simulink library "DKE_Library"  (R2018b)
settings: Solver=VariableStepAuto  StartTime=0.0  StopTime=10.0  RelTol=1e-3
undefined symbols (not defined in the file): dke, ENV, eta_panel, GM, GM_EARTH, Id, N_surf, P0_Sun, q0, r0, req_dke, RW, S_panels, S_surf, SC, v0, vf, w0, ww0, x0
libraries: MATH_library x18, ENV_Library x13, $bdroot x8, simulink x2, sharedtransform x1
(part 1 of 2)
settings Model: Creator=Andrea  LastModifiedBy=andrea

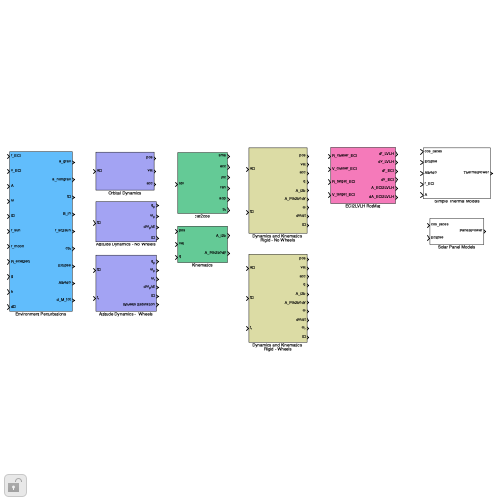
[thumbnail: Simulink's stored preview of the top-level diagram]
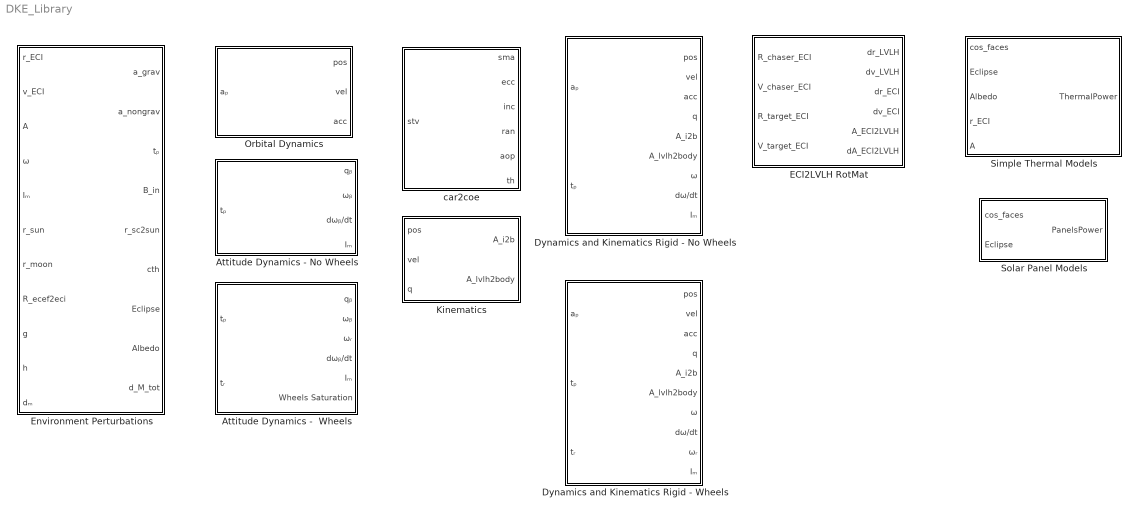
== system DKE_Library ==
  " Simple Thermal Models" : Subsystem  mask(Simple Thermal Modelling){P0_Sun=P0_Sun, BODY_RADIUS=req_dke, S_surf=S_surf, N_surf=N_surf, vf=vf}
      mask prompts: BODY_RADIUS "Earth Radius [m]:"; S_surf "Faces Areas [m²]:"; N_surf "Faces Normals:"; vf "View Factors Coefficients:"
      mask help:
      | Compute the thermal power acting on the spacecraft with a simple model.
      |
      | INPUTS:
      |   - Cosine of the angles between the surface normals and the sun direction.
      |   - Eclipse flag (1 = Eclipse ON)
      |   - Albedo falg (1 = Albedo ON)
      |   - Spacecraft Position in the Inertial Frame [m].
      |   - DCM from the inertial to the Principal Inertia Axes.
      |
      | CHANGELOG:
      |  - 2018: Andrea Colagrossi - First Release
      |  - 2023: Michele Ceresoli -  Polished
      mask DialogControl Container2 Prompt: Parameters
  Attitude Dynamics -  Wheels : Subsystem  mask(Rigid Attitude Dynamics - With Reaction Wheels){q0=q0, w0=w0, ww0=ww0, I=SC.I, invI=SC.invI, RW=RW}
      mask prompts: q0 "Initial Quaternion:"; w0 "Initial Angular Velocity [rad/s]:"; ww0 "Initial RW Angular Velocity [rad/s]"; I "Inertia Matrix [kgm²]:"; invI "Inverse Inertia Matrix [1/kgm²]"; RW "Reaction Wheels Structure:"
      mask help:
      | Integrate the controlled (with reaction wheels) attitude dynamics of a spacecraft without the flexibility and sloshing effects.
      |
      | INPUTS:
      |   - Perturbing torque [Nm]
      |   - Reaction wheels torque [Nm]
      |
      | OUTPUTS:
      |   - Quaternion from the inertial to the Principal Inertial Axes
      |   - Spacecraft angular velocity in the Principal Inertial Axes [rad/s]
      |   - Reaction wheels angular velocity [rad/s]
      |   - Angular velocity derivative in the Principal Inertial Axes [rad/s²]
      |   - Spacecraft inertia matrix [kgm²]
      |   - Wheels Saturation flag (true if saturated)
      |
      | CHANGELOG:
      |   - 2018: Andrea Colagrossi - First Release
      |   - 2023: Michele Ceresoli - Polished
      mask DialogControl Container2 Prompt: Parameters:
  Attitude Dynamics - No Wheels : Subsystem  mask(Rigid Attitude Dynamics - Without Reaction Wheels){q0=q0, w0=w0, I=SC.I, invI=SC.invI}
      mask prompts: q0 "Initial Quaternion:"; w0 "Initial Angular Velocity [rad/s]:"; I "Inertia Matrix [kgm²]:"; invI "Inverse Inertia Matrix [1/kgm²]"
      mask help:
      | Integrate the uncontrolled (no reaction wheels) attitude dynamics of a spacecraft without the flexibility and sloshing effects.
      |
      | INPUTS:
      |   - Perturbing torque [Nm]
      |
      | OUTPUTS:
      |   - Quaternion from the inertial to the Principal Inertial Axes
      |   - Spacecraft angular velocity in the Principal Inertial Axes [rad/s]
      |   - Angular velocity derivative in the Principal Inertial Axes [rad/s²]
      |   - Spacecraft inertia matrix [kgm²]
      |
      | CHANGELOG:
      |   - 2018: Andrea Colagrossi - First Release
      |   - 2023: Michele Ceresoli - Polished
      mask DialogControl Container2 Prompt: Parameters:
  Dynamics and Kinematics Rigid - No Wheels : Subsystem  mask(Rigid Dynamics and Kinematics - No Wheels){r0=r0, v0=v0, w0=w0, q0=q0, Im=SC, InvIm=SC, GM_BODY=0}
      mask prompts: r0 "Initial Position [m]:"; v0 "Initial Velocity [m/s]:"; w0 "Initial Angular velocity [rad/s]:"; q0 "Initial Quaternion:"; Im "Inertia Matrix [kgm²]"; InvIm "Inverse Inertia Matrix [1/kgm²]"; GM_BODY "Planetary Constant [m³/s²]"
      mask help:
      | Propagate the uncontrolled attitude dynamics and kinematics with a rigid model (no flexibility and sloshing).
      |
      | INPUTS:
      |   - Perturbing inertial acceleration [m/s²]
      |   - Perturbing torque in the PIA [Nm]
      |
      | OUTPUTS:
      |   - Inertial position [m]
      |   - Inertial velocity [m/s]
      |   - Inertial acceleration [m/s²]
      |   - Quaternion from the Inertial to the PIA
      |   - DCM from the Inertial to the PIA
      |   - DCM from the LVLH to the PIA
      |   - Angular velocity in the PIA [rad/s]
      |   - Angular velocity derivative in the PIA [rad/s²]
      |   - Inertia Matrix [kgm²]
      |
      | NOTES:
      |   - PIA stands for Principal Inertial Axes.
      |
      | CHANGELOG:
      |   - 2018: Andrea Colagrossi - First Release
      |   - 2023: Michele Ceresoli -  Rework, Tested and Polished
      mask DialogControl Container3 Prompt: Initial Conditions
      mask DialogControl Container4 Prompt: Properties
  Dynamics and Kinematics Rigid - Wheels : Subsystem  mask(Rigid Dynamics and Kinematics - Wheels){r0=r0, v0=v0, w0=w0, ww0=0, q0=q0, Im=SC, InvIm=ENV, GM_BODY=0, RWL=0}
      mask prompts: r0 "Initial position [m]:"; v0 "Initial velocity [m/s]:"; w0 "Initial angular velocity [rad/s]:"; ww0 "RW Initial angular velocity [rad/s]"; q0 "Initial quaternion:"; Im "Inertia Matrix [kgm²]"; InvIm "Inverse Inertia Matrix [1/kgm²]"; GM_BODY "Planetary Constant [m³/s²]"; RWL "Reaction Wheels structure"
      mask help:
      | Propagate the attitude dynamics and kinematics with a rigid model (no flexibility and sloshing) including the reaction wheels control.
      |
      | INPUTS:
      |   - Perturbing inertial acceleration [m/s²]
      |   - Perturbing torque in the PIA [Nm]
      |
      | OUTPUTS:
      |   - Inertial position [m]
      |   - Inertial velocity [m/s]
      |   - Inertial acceleration [m/s²]
      |   - Quaternion from the Inertial to the PIA
      |   - DCM from the Inertial to the PIA
      |   - DCM from the LVLH to the PIA
      |   - Angular velocity in the PIA [rad/s]
      |   - Angular velocity derivative in the PIA [rad/s²]
      |   - Reaction wheels angular velocity [rad/s]
      |   - Inertia Matrix [kgm²]
      |
      | NOTES:
      |   - PIA stands for Principal Inertial Axes.
      |
      | CHANGELOG:
      |   - 2018: Andrea Colagrossi - First Release
      |   - 2023: Michele Ceresoli -  Rework, Tested and Polished
      mask DialogControl Container3 Prompt: Initial Conditions
      mask DialogControl Container4 Prompt: Properties
  ECI2LVLH RotMat : Subsystem  mask(ECI2LVLH Rotation Block){ref_obj=1, GM=dke.GM_EARTH}
      mask prompts: ref_obj "Reference LVLH object (1 for chaser, -1 for target)"; GM "Gravitational constant [m³/s²]:"
      mask help:
      | © ASTRA - Aerospace Science and Technology Dept. - PoliMi - 2023
      |
      | Relative position and velocity rotation ECI to/from LVLH.
      |
      | Input and output in SI units [m, m/s].
      mask DialogControl Container2 Prompt: Parameters:
  Environment Perturbations : Subsystem  mask(Environment Perturbations){GM_EARTH=ENV.GM_EARTH, GM_MOON=ENV.GM_MOON, GM_SUN=ENV.GM_SUN, RADIUS_EARTH=ENV.RADIUS_EARTH, RADIUS_SUN=ENV.RADIUS_SUN, ATMO_HEIGHT=0, mag_data=ENV.mag_data, grav_data=ENV.grav_data, rho_h=ENV.rho_h, NS=SC.NS, S_faces=SC.S_surf, N_faces=SC.N_surf, R_faces=SC.R_surf, c_dif=SC.c_dif, c_spe=SC.c_spe, CD=SC.C_D, mass=SC.m_sc, paras_dipole=SC.d, Keddy=SC.Keddy}
      mask prompts: GM_EARTH "Earth's Gravitational Constant [m³/s²]:"; GM_MOON "Moon's Gravitational Constant [m³/s²]:"; GM_SUN "Sun's Gravitational Constant [m³/s²]:"; RADIUS_EARTH "Earth's Radius [m]"; RADIUS_SUN "Sun's Radius [m]"; ATMO_HEIGHT "Earth's Atmosphere Height [m]"; mag_data "Magnetic Field Data:"; grav_data "Gravity Field Data:"; rho_h "Air Density Data:"; NS "Number of Faces"; S_faces "Faces Areas [m²]:"; N_faces "Faces Normals:"; R_faces "Faces Center of Pressures wrt CoM [m]:"; c_dif "Diffuse Coefficient [-]:"; c_spe "Specular Coefficient [-]:"; CD "Drag Coefficient [-]:"; mass "Mass [kg]:"; paras_dipole "Parasitic Magnetic Dipole [Am²]:"; Keddy "Eddy Currents Coefficient []:"
      mask help:
      | Compute the environment perturbing acceleration [m/s²] and torque [Nm] that act on a spacecraft. The perturbations include:
      |   - Moon's gravity
      |   - Sun's gravity
      |   - Earth's spherical harmonics
      |   - Gravity gradient torque
      |   - SRP acceleration and torque (with the plate model)
      |   - Drag acceleration and torque (with the plate model)
      |   - Magnetic torque (dipole and Eddy currents)
      |
      | INPUTS:
      |   - r_ECI, v_ECI: Spacecraft positions in the ECI frame [m]
      |   - A: DCM from the inertial to the Principal Inertia Frame
      |   - ω: Spacecraft angular velocity in the Principal Inertia Frame [rad/s]
      |   - Iₘ: Spacecraft Inertia Matrix [kgm²]
      |   - TT: Terrestrial time seconds since J2000
      |   - r_sun, r_moon: Sun's and Moon's positions in the ECI frame [m]
      |   - R_ecef2eci: ECEF to ECI rotation matrix
      |   - g, h: Magnetic Field coefficients at epoch.
      |   - dₘ: Magnetorquer Magnetic Dipole [Am²]
      |
      | NOTES:
      |   - A simple atmospheric model is used to compute the air density.
      |   - The gravity field data is extracted from the "load_gravity_model" function.
      |   - All the inputs and outputs are expressed in SI units (m, m/s, rad/s, kg, T, etc..).
      |
      | CHANGELOG:
      |   - 2018: Andrea Colagrossi - First Release
      |   - 2023: Michele Ceresoli - Rework, Testing and Polishing
      mask DialogControl Container3 Prompt: Environment:
      mask DialogControl Container4 Prompt: Spacecraft Geometry
      mask DialogControl Container5 Prompt: Spacecraft Properties
  Kinematics : Subsystem  mask(Kinematics){GM_BODY=0}
      mask prompts: GM_BODY "Planetary Gravitational Constant [m³/s²]:"
      mask help:
      | Compute the LVLH to Body and Inertial to Body 3x3 rotation matrices.
      |
      | INPUTS:
      |   - Attitude quaternion from the inertial to the body frame.
      |   - Inertial position [m]
      |   - Inertial velocity [m/s]
      |
      | CHANGELOG:
      |   - 2018: Andrea Colagrossi/Lorenzo Bucci - First Release
      |   - 2023: Michele Ceresoli - Reworked, Tested and Polished
  Orbital Dynamics : Subsystem  mask(Orbital Dynamics){r0=x0, v0=v0, GM=GM}
      mask prompts: r0 "Initial Position [m]:"; v0 "Initial Velocity [m/s]:"; GM "Central Body Gravitational Constant [m³/s²]:"
      mask help:
      | Propagate the spacecraft orbital dynamics by including the input perturbing acceleration to the two-body gravitational acceleration.
      |
      | INPUTS:
      |  - Perturbing acceleration [m/s²]
      |
      | OUTPUTS:
      |  - Inertial Position [m]
      |  - Inertial Velocity [m/s]
      |  - Inertial Acceleration [m/s²]
      |
      | CHANGELOG:
      |  - 2018: Andrea Colagrossi - First Release
      |  - 2023: Michele Ceresoli - Testing and Polishing
  Solar Panel Models : Subsystem  mask{P0_Sun=P0_Sun, eta_panel=eta_panel, Id=Id, S_panels=S_panels}
      mask help:
      | © Andrea Colagrossi - Aerospace Science and Technology Dept. - PoliMi - 2018
      |
      | Panels Electric Modelling
      |
      | Input and output in SI units [m, m/s, rad/s, kg, T, etc.]
      |
      | Cos_faces: Cosine of the Sun on Spacecraft Surfaces
      | Eclipse: Flag of the Eclipse Status (1 = Eclipse ON)
  car2coe : Subsystem  mask(Cartesian to Classical Orbital Elements (COE)){GM=GM_EARTH}
      mask prompts: GM "Planetary Gravitational Constant:"
      mask help: Convert a Cartesian state (position and velocity) to the Classical Orbital Elements (COE).

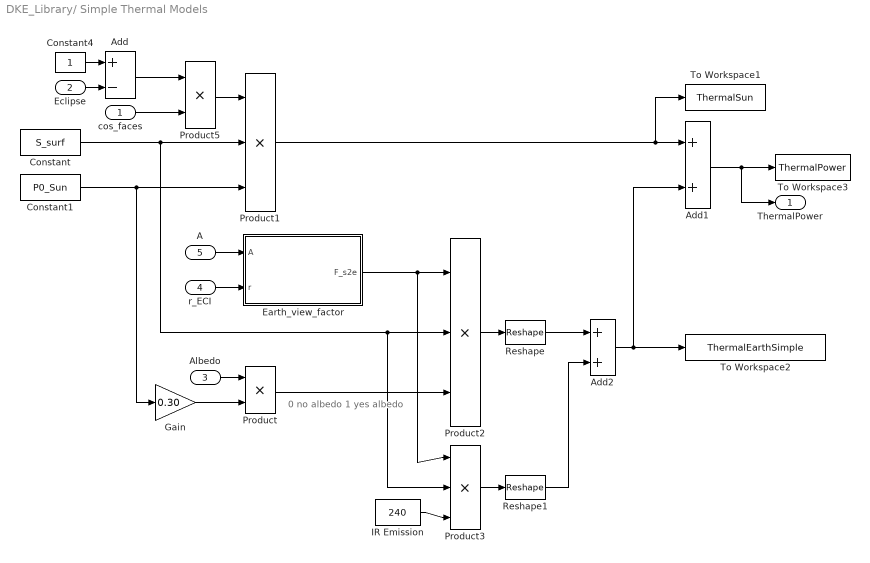
== system DKE_Library/ Simple Thermal Models ==
  note: 0 no albedo
      | 1 yes albedo
  cos_faces : Inport
  Eclipse : Inport  Port=2
  Albedo : Inport  Port=3
  r_ECI : Inport  Port=4
  A : Inport  Port=5
  Add : Sum  Inputs=+-
  Add1 : Sum
  Add2 : Sum
  Constant : Constant  Value=S_surf
  Constant1 : Constant  Value=P0_Sun
  Constant4 : Constant
  "Earth_view_factor " : Subsystem
  Gain : Gain  Gain=0.30
  IR Emission : Constant  Value=240
  Product : Product
  Product1 : Product  Inputs=3
  Product2 : Product  Inputs=3
  Product3 : Product  Inputs=3
  Product5 : Product
  Reshape : Reshape
  Reshape1 : Reshape
  To Workspace1 : ToWorkspace  VariableName=ThermalSun  SampleTime=-1
  To Workspace2 : ToWorkspace  VariableName=ThermalEarthSimple  SampleTime=-1
  To Workspace3 : ToWorkspace  VariableName=ThermalPower  SampleTime=-1
  ThermalPower : Outport  VectorParamsAs1DForOutWhenUnconnected=off
  wires:
  Gain/1 -> Product/2
  Albedo/1 -> Product/1
  Product/1 -> Product2/3
  IR Emission/1 -> Product3/3
  Constant1/1 -> Product1/3, Gain/1
  Product1/1 -> To Workspace1/1, Add1/1
  Product3/1 -> Reshape1/1
  Product2/1 -> Reshape/1
  Product5/1 -> Product1/1
  Eclipse/1 -> Add/2
  Constant4/1 -> Add/1
  cos_faces/1 -> Product5/2
  Add/1 -> Product5/1
  Constant/1 -> Product1/2, Product3/2, Product2/2
  Add2/1 -> To Workspace2/1, Add1/2
  Reshape/1 -> Add2/1
  Reshape1/1 -> Add2/2
  "Earth_view_factor "/1(F_s2e) -> Product2/1, Product3/1
  A/1 -> "Earth_view_factor "/1(A)
  r_ECI/1 -> "Earth_view_factor "/2("r ")
  Add1/1 -> ThermalPower/1, To Workspace3/1

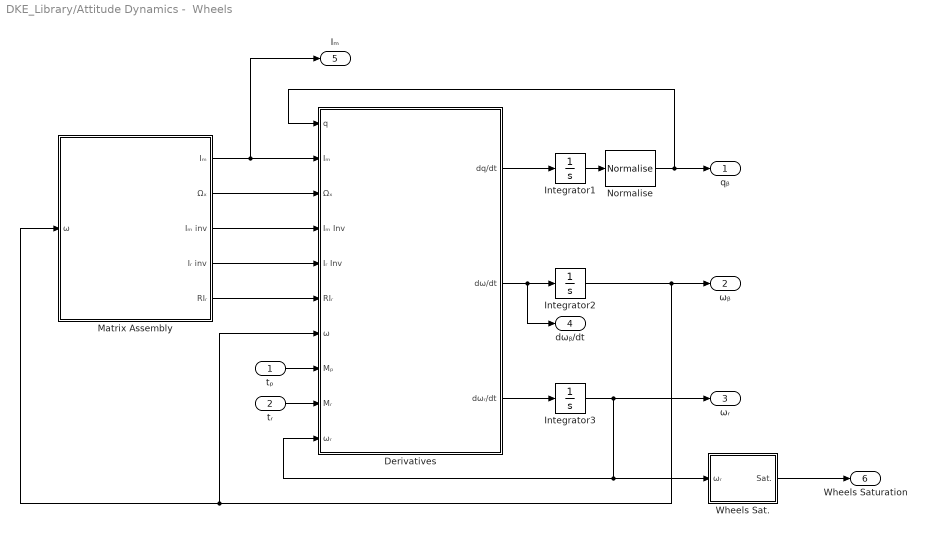
== system DKE_Library/Attitude Dynamics -  Wheels ==
  tₚ : Inport
  tᵣ : Inport  Port=2
  Derivatives : Subsystem
  Integrator1 : Integrator  InitialCondition=q0
  Integrator2 : Integrator  InitialCondition=w0
  Integrator3 : Integrator  InitialCondition=ww0  LimitOutput=on  UpperSaturationLimit=RW.MaxWheelW  LowerSaturationLimit=-RW.MaxWheelW
  Matrix Assembly : Subsystem
  Normalise : MATH_library/Normalise
  Wheels Sat. : Subsystem
  qᵦ : Outport  VectorParamsAs1DForOutWhenUnconnected=off
  ωᵦ : Outport  Port=2  VectorParamsAs1DForOutWhenUnconnected=off
  ωᵣ : Outport  Port=3  VectorParamsAs1DForOutWhenUnconnected=off
  dωᵦ/dt : Outport  Port=4  VectorParamsAs1DForOutWhenUnconnected=off
  Iₘ : Outport  Port=5  VectorParamsAs1DForOutWhenUnconnected=off
  Wheels Saturation : Outport  Port=6  VectorParamsAs1DForOutWhenUnconnected=off
  wires:
  Matrix Assembly/3(Iₘ inv) -> Derivatives/4(Iₘ Inv)
  Derivatives/2(dω/dt) -> dωᵦ/dt/1, Integrator2/1
  tₚ/1 -> Derivatives/8(Mₚ)
  Integrator2/1 -> ωᵦ/1, Derivatives/7(ω), Matrix Assembly/1("ω ")
  Matrix Assembly/1("Iₘ ") -> Derivatives/2(Iₘ), Iₘ/1
  Matrix Assembly/2(Ωₓ) -> Derivatives/3(Ωₓ)
  Derivatives/1(dq/dt) -> Integrator1/1
  Integrator1/1 -> Normalise/1
  Normalise/1 -> qᵦ/1, Derivatives/1(q)
  tᵣ/1 -> Derivatives/9(Mᵣ)
  Matrix Assembly/5(RIᵣ) -> Derivatives/6(RIᵣ)
  Matrix Assembly/4(Iᵣ inv) -> Derivatives/5(Iᵣ Inv)
  Derivatives/3(dωᵣ/dt) -> Integrator3/1
  Integrator3/1 -> Wheels Sat./1(ωᵣ), Derivatives/10(ωᵣ), ωᵣ/1
  Wheels Sat./1(Sat.) -> Wheels Saturation/1

== system DKE_Library/Attitude Dynamics - No Wheels ==
  tₚ : Inport
  Derivatives : Subsystem
  Integrator1 : Integrator  InitialCondition=q0
  Integrator2 : Integrator  InitialCondition=w0
  Matrix Assembly : Subsystem
  Normalise : MATH_library/Normalise
  qᵦ : Outport  VectorParamsAs1DForOutWhenUnconnected=off
  ωᵦ : Outport  Port=2  VectorParamsAs1DForOutWhenUnconnected=off
  dωᵦ/dt : Outport  Port=3  VectorParamsAs1DForOutWhenUnconnected=off
  Iₘ : Outport  Port=4  VectorParamsAs1DForOutWhenUnconnected=off
  wires:
  Matrix Assembly/3(Iₘ inv) -> Derivatives/4(Iₘ Inv)
  Derivatives/2(dω/dt) -> dωᵦ/dt/1, Integrator2/1
  tₚ/1 -> Derivatives/6(tₚ)
  Integrator2/1 -> ωᵦ/1, Derivatives/5(ω), Matrix Assembly/1("ω ")
  Matrix Assembly/1("Iₘ ") -> Iₘ/1, Derivatives/2(Iₘ)
  Matrix Assembly/2(Ωₓ) -> Derivatives/3(Ωₓ)
  Derivatives/1(dq/dt) -> Integrator1/1
  Integrator1/1 -> Normalise/1
  Normalise/1 -> qᵦ/1, Derivatives/1(q)

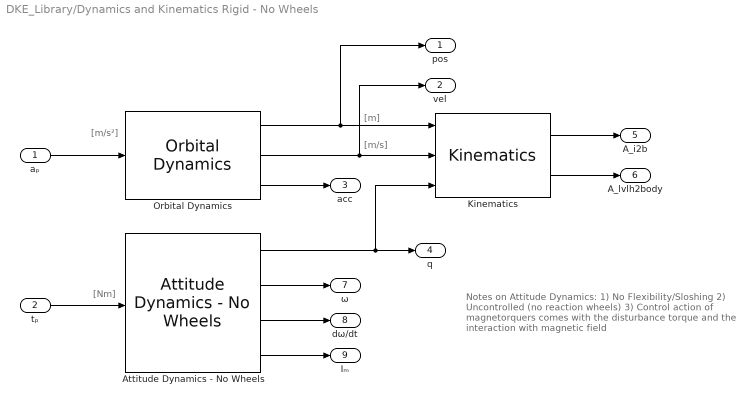
== system DKE_Library/Dynamics and Kinematics Rigid - No Wheels ==
  note: [m/s²]
  note: [Nm]
  note: [m]
  note: [m/s]
  note: Notes on Attitude Dynamics:
      | 1) No Flexibility/Sloshing
      | 2) Uncontrolled (no reaction wheels)
      | 3) Control action of magnetorquers comes with the disturbance torque and the interaction with magnetic field
  aₚ : Inport
  tₚ : Inport  Port=2
  Attitude Dynamics - No Wheels : $bdroot/Attitude Dynamics - No Wheels  q0=q0  w0=w0  I=Im  invI=InvIm
  Kinematics : $bdroot/Kinematics  GM_BODY=GM_BODY
  Orbital Dynamics : $bdroot/Orbital Dynamics  r0=r0  v0=v0  GM=GM_BODY
  pos : Outport  VectorParamsAs1DForOutWhenUnconnected=off
  vel : Outport  Port=2  VectorParamsAs1DForOutWhenUnconnected=off
  acc : Outport  Port=3  VectorParamsAs1DForOutWhenUnconnected=off
  q : Outport  Port=4  VectorParamsAs1DForOutWhenUnconnected=off
  A_i2b : Outport  Port=5  VectorParamsAs1DForOutWhenUnconnected=off
  A_lvlh2body : Outport  Port=6  VectorParamsAs1DForOutWhenUnconnected=off
  ω : Outport  Port=7  VectorParamsAs1DForOutWhenUnconnected=off
  dω/dt : Outport  Port=8  VectorParamsAs1DForOutWhenUnconnected=off
  Iₘ : Outport  Port=9  VectorParamsAs1DForOutWhenUnconnected=off
  wires:
  Orbital Dynamics/1 -> pos/1, Kinematics/1
  aₚ/1 -> Orbital Dynamics/1
  Kinematics/1 -> A_i2b/1
  Attitude Dynamics - No Wheels/1 -> q/1, Kinematics/3
  Orbital Dynamics/2 -> vel/1, Kinematics/2
  Orbital Dynamics/3 -> acc/1
  Attitude Dynamics - No Wheels/2 -> ω/1
  Kinematics/2 -> A_lvlh2body/1
  tₚ/1 -> Attitude Dynamics - No Wheels/1
  Attitude Dynamics - No Wheels/3 -> dω/dt/1
  Attitude Dynamics - No Wheels/4 -> Iₘ/1

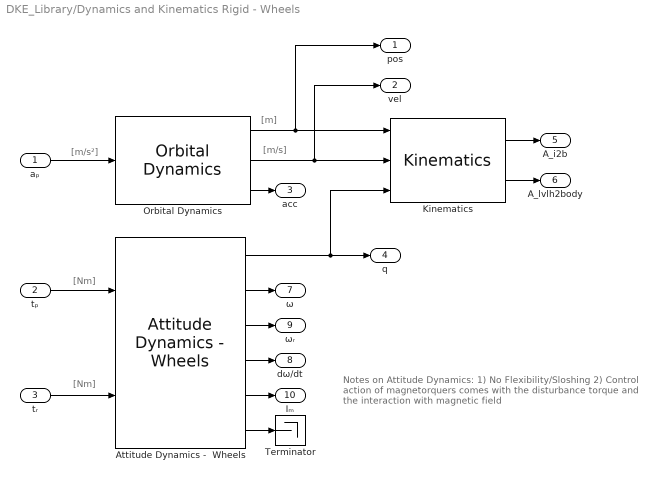
== system DKE_Library/Dynamics and Kinematics Rigid - Wheels ==
  note: [m/s²]
  note: [Nm]
  note: [m]
  note: [m/s]
  note: [Nm]
  note: Notes on Attitude Dynamics:
      | 1) No Flexibility/Sloshing
      | 2) Control action of magnetorquers comes with the disturbance torque and the interaction with magnetic field
  aₚ : Inport
  tₚ : Inport  Port=2
  tᵣ : Inport  Port=3
  Attitude Dynamics -  Wheels : $bdroot/Attitude Dynamics -  Wheels  q0=q0  w0=w0  ww0=ww0  I=Im  invI=InvIm  RW=RWL
  Kinematics : $bdroot/Kinematics  GM_BODY=GM_BODY
  Orbital Dynamics : $bdroot/Orbital Dynamics  r0=r0  v0=v0  GM=GM_BODY
  Terminator : Terminator
  pos : Outport  VectorParamsAs1DForOutWhenUnconnected=off
  vel : Outport  Port=2  VectorParamsAs1DForOutWhenUnconnected=off
  acc : Outport  Port=3  VectorParamsAs1DForOutWhenUnconnected=off
  q : Outport  Port=4  VectorParamsAs1DForOutWhenUnconnected=off
  A_i2b : Outport  Port=5  VectorParamsAs1DForOutWhenUnconnected=off
  A_lvlh2body : Outport  Port=6  VectorParamsAs1DForOutWhenUnconnected=off
  ω : Outport  Port=7  VectorParamsAs1DForOutWhenUnconnected=off
  dω/dt : Outport  Port=8  VectorParamsAs1DForOutWhenUnconnected=off
  ωᵣ : Outport  Port=9  VectorParamsAs1DForOutWhenUnconnected=off
  Iₘ : Outport  Port=10  VectorParamsAs1DForOutWhenUnconnected=off
  wires:
  Orbital Dynamics/1 -> pos/1, Kinematics/1
  aₚ/1 -> Orbital Dynamics/1
  Kinematics/1 -> A_i2b/1
  Attitude Dynamics -  Wheels/1 -> q/1, Kinematics/3
  Orbital Dynamics/2 -> vel/1, Kinematics/2
  Orbital Dynamics/3 -> acc/1
  Attitude Dynamics -  Wheels/2 -> ω/1
  Kinematics/2 -> A_lvlh2body/1
  tₚ/1 -> Attitude Dynamics -  Wheels/1
  tᵣ/1 -> Attitude Dynamics -  Wheels/2
  Attitude Dynamics -  Wheels/6 -> Terminator/1
  Attitude Dynamics -  Wheels/5 -> Iₘ/1
  Attitude Dynamics -  Wheels/4 -> dω/dt/1
  Attitude Dynamics -  Wheels/3 -> ωᵣ/1

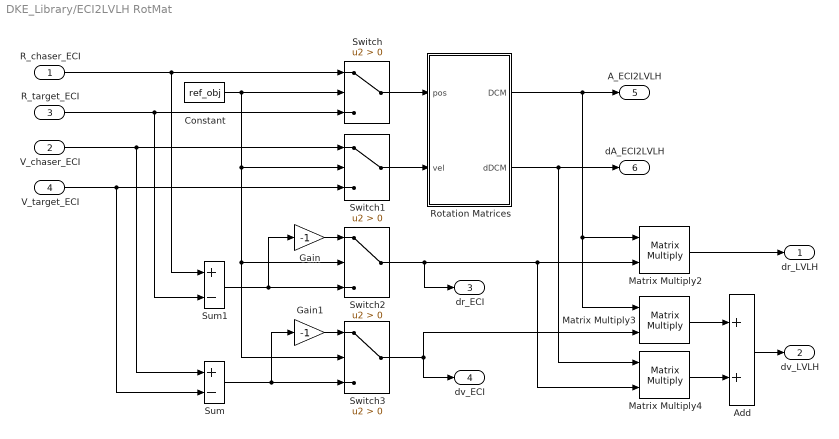
== system DKE_Library/ECI2LVLH RotMat ==
  R_chaser_ECI : Inport
  V_chaser_ECI : Inport  Port=2
  R_target_ECI : Inport  Port=3
  V_target_ECI : Inport  Port=4
  Add : Sum
  Constant : Constant  Value=ref_obj
  Gain : Gain  Gain=-1
  Gain1 : Gain  Gain=-1
  Matrix Multiply2 : Product  Multiplication=Matrix(*)
  Matrix Multiply3 : Product  Multiplication=Matrix(*)
  Matrix Multiply4 : Product  Multiplication=Matrix(*)
  Rotation Matrices : Subsystem
  Sum : Sum  Inputs=+-
  Sum1 : Sum  Inputs=+-
  Switch{,1..3} (4 alike) : Switch  Criteria=u2 > Threshold
  dr_LVLH : Outport  VectorParamsAs1DForOutWhenUnconnected=off
  dv_LVLH : Outport  Port=2  VectorParamsAs1DForOutWhenUnconnected=off
  dr_ECI : Outport  Port=3  VectorParamsAs1DForOutWhenUnconnected=off
  dv_ECI : Outport  Port=4  VectorParamsAs1DForOutWhenUnconnected=off
  A_ECI2LVLH : Outport  Port=5  VectorParamsAs1DForOutWhenUnconnected=off
  dA_ECI2LVLH : Outport  Port=6  VectorParamsAs1DForOutWhenUnconnected=off
  wires:
  R_target_ECI/1 -> Switch/3, Sum1/2
  R_chaser_ECI/1 -> Sum1/1, Switch/1
  Sum1/1 -> Gain/1, Switch2/3
  Gain/1 -> Switch2/1
  Switch2/1 -> Matrix Multiply4/2, Matrix Multiply2/2, dr_ECI/1
  Gain1/1 -> Switch3/1
  Sum/1 -> Switch3/3, Gain1/1
  Switch3/1 -> Matrix Multiply3/2, dv_ECI/1
  Constant/1 -> Switch2/2, Switch3/2, Switch1/2, Switch/2
  V_chaser_ECI/1 -> Sum/1, Switch1/1
  V_target_ECI/1 -> Sum/2, Switch1/3
  Switch/1 -> Rotation Matrices/1(pos)
  Switch1/1 -> Rotation Matrices/2(vel)
  Rotation Matrices/1(DCM) -> A_ECI2LVLH/1, Matrix Multiply2/1, Matrix Multiply3/1
  Matrix Multiply2/1 -> dr_LVLH/1
  Matrix Multiply3/1 -> Add/1
  Matrix Multiply4/1 -> Add/2
  Rotation Matrices/2(dDCM) -> dA_ECI2LVLH/1, Matrix Multiply4/1
  Add/1 -> dv_LVLH/1

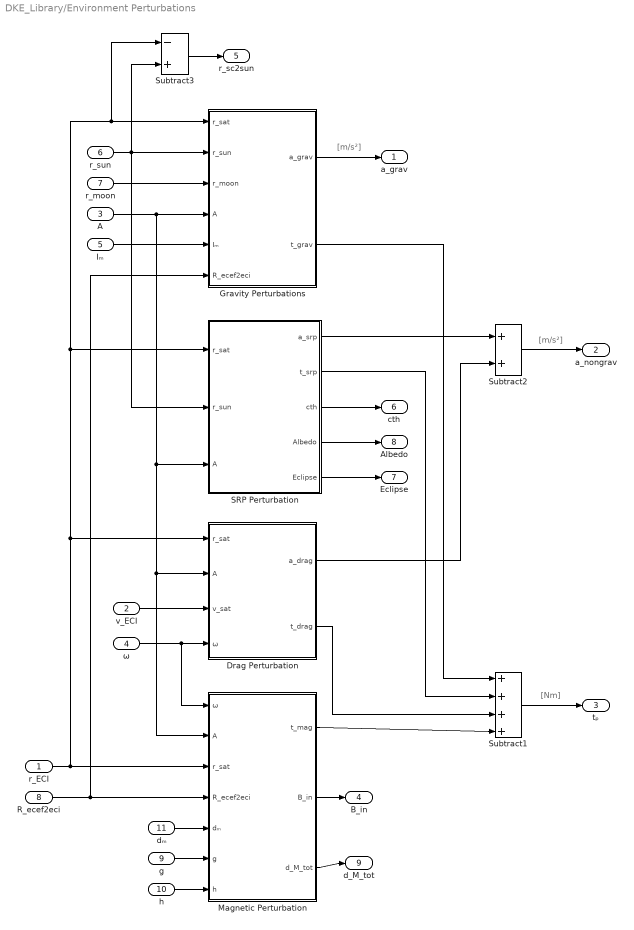
== system DKE_Library/Environment Perturbations ==
  note: [m/s²]
  note: [Nm]
  note: [m/s²]
  r_ECI : Inport
  v_ECI : Inport  Port=2
  A : Inport  Port=3
  ω : Inport  Port=4
  Iₘ : Inport  Port=5
  r_sun : Inport  Port=6
  r_moon : Inport  Port=7
  R_ecef2eci : Inport  Port=8
  g : Inport  Port=9
  h : Inport  Port=10
  dₘ : Inport  Port=11
  Drag Perturbation : Subsystem
  Gravity Perturbations : Subsystem
  Magnetic Perturbation : Subsystem
  SRP Perturbation : Subsystem
  Subtract1 : Sum  Inputs=++++
  Subtract2 : Sum
  Subtract3 : Sum  Inputs=-+
  a_grav : Outport  VectorParamsAs1DForOutWhenUnconnected=off
  a_nongrav : Outport  Port=2  VectorParamsAs1DForOutWhenUnconnected=off
  tₚ : Outport  Port=3  VectorParamsAs1DForOutWhenUnconnected=off
  B_in : Outport  Port=4  VectorParamsAs1DForOutWhenUnconnected=off
  r_sc2sun : Outport  Port=5  VectorParamsAs1DForOutWhenUnconnected=off
  cth : Outport  Port=6  VectorParamsAs1DForOutWhenUnconnected=off
  Eclipse : Outport  Port=7  VectorParamsAs1DForOutWhenUnconnected=off
  Albedo : Outport  Port=8  VectorParamsAs1DForOutWhenUnconnected=off
  d_M_tot : Outport  Port=9  VectorParamsAs1DForOutWhenUnconnected=off
  wires:
  Subtract1/1 -> tₚ/1
  Drag Perturbation/2(t_drag) -> Subtract1/3
  ω/1 -> Magnetic Perturbation/1(ω), Drag Perturbation/4(ω)
  SRP Perturbation/3(cth) -> cth/1
  v_ECI/1 -> Drag Perturbation/3(v_sat)
  Gravity Perturbations/2(t_grav) -> Subtract1/1
  A/1 -> Gravity Perturbations/4(A), Drag Perturbation/2(A), Magnetic Perturbation/2(A), SRP Perturbation/3(A)
  Iₘ/1 -> Gravity Perturbations/5(Iₘ)
  Magnetic Perturbation/1(t_mag) -> Subtract1/4
  r_moon/1 -> Gravity Perturbations/3(r_moon)
  g/1 -> Magnetic Perturbation/6(g)
  r_sun/1 -> Gravity Perturbations/2(r_sun), Subtract3/2, SRP Perturbation/2(r_sun)
  dₘ/1 -> Magnetic Perturbation/5(dₘ)
  SRP Perturbation/2(t_srp) -> Subtract1/2
  Gravity Perturbations/1(a_grav) -> a_grav/1
  R_ecef2eci/1 -> Gravity Perturbations/6(R_ecef2eci), Magnetic Perturbation/4(R_ecef2eci)
  r_ECI/1 -> Gravity Perturbations/1(r_sat), Subtract3/1, SRP Perturbation/1(r_sat), Drag Perturbation/1(r_sat), Magnetic Perturbation/3(r_sat)
  Magnetic Perturbation/2(B_in) -> B_in/1
  SRP Perturbation/4(Albedo) -> Albedo/1
  SRP Perturbation/5(Eclipse) -> Eclipse/1
  Magnetic Perturbation/3(d_M_tot) -> d_M_tot/1
  Subtract2/1 -> a_nongrav/1
  SRP Perturbation/1(a_srp) -> Subtract2/1
  Drag Perturbation/1(a_drag) -> Subtract2/2
  Subtract3/1 -> r_sc2sun/1
  h/1 -> Magnetic Perturbation/7(h)

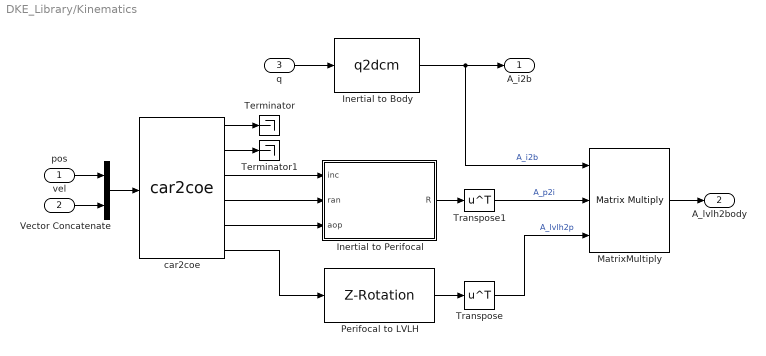
== system DKE_Library/Kinematics ==
  pos : Inport
  vel : Inport  Port=2
  q : Inport  Port=3
  Inertial to Body : MATH_library/q2dcm
  Inertial to Perifocal : Subsystem
  MatrixMultiply : Product  Inputs=3  Multiplication=Matrix(*)
  Perifocal to LVLH : MATH_library/Z-Rotation
  Terminator : Terminator
  Terminator1 : Terminator
  Transpose : Math  Operator=transpose  SaturateOnIntegerOverflow=on
  Transpose1 : Math  Operator=transpose  SaturateOnIntegerOverflow=on
  Vector Concatenate : Concatenate
  car2coe : $bdroot/car2coe  GM=GM_BODY
  A_i2b : Outport  VectorParamsAs1DForOutWhenUnconnected=off
  A_lvlh2body : Outport  Port=2  VectorParamsAs1DForOutWhenUnconnected=off
  wires:
  q/1 -> Inertial to Body/1
  Inertial to Body/1 -> MatrixMultiply/1, A_i2b/1  "A_i2b"
  pos/1 -> Vector Concatenate/1
  Vector Concatenate/1 -> car2coe/1
  vel/1 -> Vector Concatenate/2
  car2coe/1 -> Terminator/1
  car2coe/2 -> Terminator1/1
  car2coe/3 -> Inertial to Perifocal/1(inc)
  car2coe/4 -> Inertial to Perifocal/2(ran)
  car2coe/5 -> Inertial to Perifocal/3(aop)
  car2coe/6 -> Perifocal to LVLH/1
  Perifocal to LVLH/1 -> Transpose/1
  Transpose/1 -> MatrixMultiply/3  "A_lvlh2p"
  Inertial to Perifocal/1(R) -> Transpose1/1
  Transpose1/1 -> MatrixMultiply/2  "A_p2i"
  MatrixMultiply/1 -> A_lvlh2body/1

== system DKE_Library/Orbital Dynamics ==
  note: [m/s²]
  note: d²r/dt²
  note: dr/dt
  note: [m/s]
  note: [m]
  "aₚ " : Inport
  Integrator : Integrator  InitialCondition=v0
  Integrator1 : Integrator  InitialCondition=r0
  Sum1 : Sum  Inputs=|++
  Two-Body Gravity : ENV_Library/Two-Body Gravity  GM=GM
  pos : Outport  VectorParamsAs1DForOutWhenUnconnected=off
  vel : Outport  Port=2  VectorParamsAs1DForOutWhenUnconnected=off
  acc : Outport  Port=3  VectorParamsAs1DForOutWhenUnconnected=off
  wires:
  Two-Body Gravity/1 -> Sum1/2
  "aₚ "/1 -> Sum1/1
  Sum1/1 -> Integrator/1, acc/1
  Integrator/1 -> vel/1, Integrator1/1
  Integrator1/1 -> pos/1, Two-Body Gravity/1  "r"

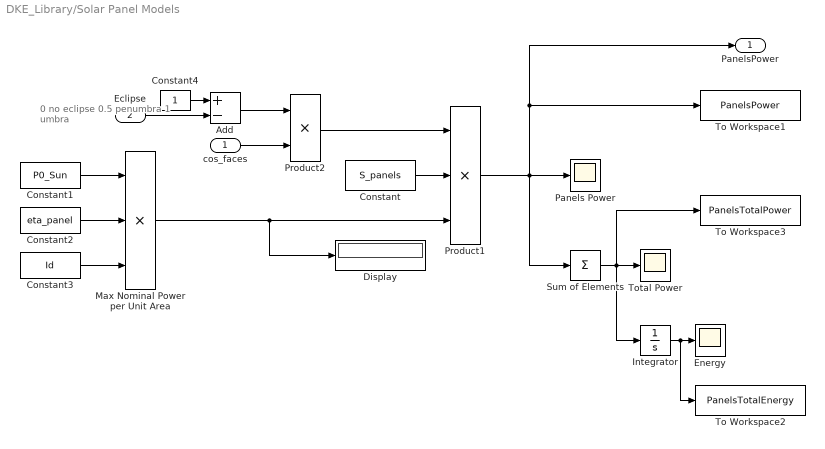
== system DKE_Library/Solar Panel Models ==
  note: 0 no eclipse
      | 0.5 penumbra
      | 1 umbra
  cos_faces : Inport
  "Eclipse " : Inport  Port=2
  Add : Sum  Inputs=+-
  Constant : Constant  Value=S_panels
  Constant1 : Constant  Value=P0_Sun
  Constant2 : Constant  Value=eta_panel
  Constant3 : Constant  Value=Id
  Constant4 : Constant
  Display : Display
  Energy : Scope
  Integrator : Integrator
  Max Nominal Power per Unit Area : Product  Inputs=3
  Panels Power : Scope
  Product1 : Product  Inputs=3
  Product2 : Product
  Sum of Elements : Sum  Inputs=+
  To Workspace1 : ToWorkspace  VariableName=PanelsPower  SampleTime=-1
  To Workspace2 : ToWorkspace  VariableName=PanelsTotalEnergy  SampleTime=-1
  To Workspace3 : ToWorkspace  VariableName=PanelsTotalPower  SampleTime=-1
  Total Power : Scope
  PanelsPower : Outport  VectorParamsAs1DForOutWhenUnconnected=off
  wires:
  Integrator/1 -> Energy/1, To Workspace2/1
  Sum of Elements/1 -> Total Power/1, Integrator/1, To Workspace3/1
  Constant/1 -> Product1/2
  Max Nominal Power per Unit Area/1 -> Product1/3, Display/1
  Constant3/1 -> Max Nominal Power per Unit Area/3
  Constant1/1 -> Max Nominal Power per Unit Area/1
  Constant2/1 -> Max Nominal Power per Unit Area/2
  cos_faces/1 -> Product2/2
  Product1/1 -> Panels Power/1, PanelsPower/1, To Workspace1/1, Sum of Elements/1
  "Eclipse "/1 -> Add/2
  Constant4/1 -> Add/1
  Add/1 -> Product2/1
  Product2/1 -> Product1/1

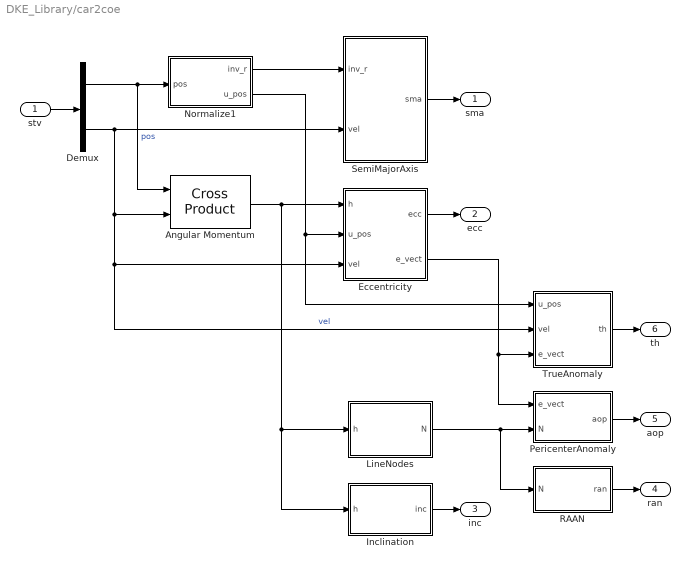
== system DKE_Library/car2coe ==
  stv : Inport
  Angular Momentum : MATH_library/Cross Product
  Demux : Demux  Outputs=2
  Eccentricity : Subsystem
  Inclination : Subsystem
  LineNodes : Subsystem
  Normalize1 : Subsystem
  PericenterAnomaly : Subsystem
  RAAN : Subsystem
  SemiMajorAxis : Subsystem
  TrueAnomaly : Subsystem
  sma : Outport  VectorParamsAs1DForOutWhenUnconnected=off
  ecc : Outport  Port=2  VectorParamsAs1DForOutWhenUnconnected=off
  inc : Outport  Port=3  VectorParamsAs1DForOutWhenUnconnected=off
  ran : Outport  Port=4  VectorParamsAs1DForOutWhenUnconnected=off
  aop : Outport  Port=5  VectorParamsAs1DForOutWhenUnconnected=off
  th : Outport  Port=6  VectorParamsAs1DForOutWhenUnconnected=off
  wires:
  Normalize1/2(u_pos) -> TrueAnomaly/1(u_pos), Eccentricity/2(u_pos)
  Normalize1/1(inv_r) -> SemiMajorAxis/1(inv_r)
  Eccentricity/2(e_vect) -> TrueAnomaly/3(e_vect), PericenterAnomaly/1(e_vect)
  Angular Momentum/1 -> LineNodes/1(h), Inclination/1(h), Eccentricity/1(h)
  Eccentricity/1(ecc) -> ecc/1
  stv/1 -> Demux/1
  Demux/2 -> TrueAnomaly/2(vel), Eccentricity/3(vel), Angular Momentum/2, SemiMajorAxis/2(vel)  "vel"
  Demux/1 -> Angular Momentum/1, Normalize1/1(pos)  "pos"
  LineNodes/1(N) -> PericenterAnomaly/2(N), RAAN/1(N)
  SemiMajorAxis/1(sma) -> sma/1
  Inclination/1(inc) -> inc/1
  RAAN/1(ran) -> ran/1
  PericenterAnomaly/1(aop) -> aop/1
  TrueAnomaly/1(th) -> th/1

== system DKE_Library/ Simple Thermal Models/Earth_view_factor  ==
  A : Inport
  "r " : Inport  Port=2
  -r : Gain  Gain=-1
  Acos : Trigonometry  Operator=acos
  Divide : Product  Inputs=*/
  Earth radius [m] : Constant  Value=BODY_RADIUS
  Nadir Vector in B : Product  Multiplication=Matrix(*)
  Subtract : Sum  Inputs=+-
  Vector Cos Angle w.r.t S/C Faces : Subsystem
  Vector Norm : MATH_library/Vector Norm
  from rad to deg : Gain  Gain=180/pi
  n-D Lookup Table : Lookup_n-D  BreakpointsForDimension1=vf.bp1  BreakpointsForDimension2=vf.bp2  BreakpointsForDimension3=[5, 7]  Table=vf.table  InternalRulePriority=Speed  RndMeth=Simplest  InputSameDT=on
  F_s2e : Outport  VectorParamsAs1DForOutWhenUnconnected=off
  wires:
  n-D Lookup Table/1 -> F_s2e/1
  Nadir Vector in B/1 -> Vector Cos Angle w.r.t S/C Faces/1(vect)
  A/1 -> Nadir Vector in B/1
  Subtract/1 -> Divide/1  "z orbit"
  Vector Cos Angle w.r.t S/C Faces/1(cos_f) -> Acos/1
  -r/1 -> Nadir Vector in B/2
  "r "/1 -> Vector Norm/1, -r/1
  Acos/1 -> from rad to deg/1
  Divide/1 -> n-D Lookup Table/1  "z/R"
  from rad to deg/1 -> n-D Lookup Table/2
  Earth radius [m]/1 -> Divide/2, Subtract/2
  Vector Norm/1 -> Subtract/1  "r"

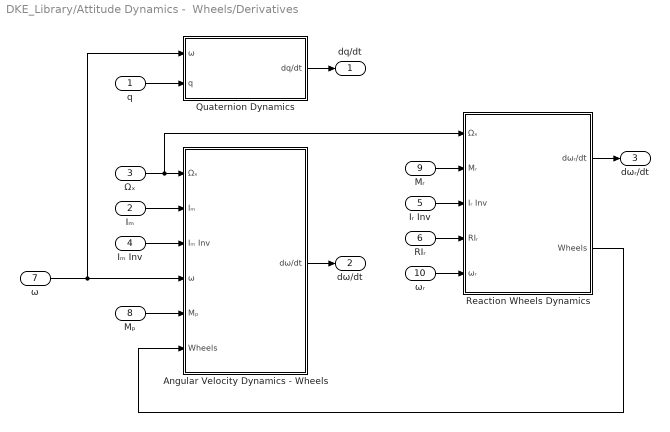
== system DKE_Library/Attitude Dynamics -  Wheels/Derivatives ==
  q : Inport
  Iₘ : Inport  Port=2
  Ωₓ : Inport  Port=3
  Iₘ Inv : Inport  Port=4
  Iᵣ Inv : Inport  Port=5
  RIᵣ : Inport  Port=6
  ω : Inport  Port=7
  Mₚ : Inport  Port=8
  Mᵣ : Inport  Port=9
  ωᵣ : Inport  Port=10
  Angular Velocity Dynamics - Wheels : Subsystem
  Quaternion Dynamics : Subsystem
  Reaction Wheels Dynamics : Subsystem
  dq/dt : Outport  VectorParamsAs1DForOutWhenUnconnected=off
  dω/dt : Outport  Port=2  VectorParamsAs1DForOutWhenUnconnected=off
  dωᵣ/dt : Outport  Port=3  VectorParamsAs1DForOutWhenUnconnected=off
  wires:
  Mₚ/1 -> Angular Velocity Dynamics - Wheels/5(Mₚ)
  Iₘ Inv/1 -> Angular Velocity Dynamics - Wheels/3(Iₘ Inv)
  Angular Velocity Dynamics - Wheels/1(dω/dt) -> dω/dt/1
  Iₘ/1 -> Angular Velocity Dynamics - Wheels/2(Iₘ)
  ω/1 -> Angular Velocity Dynamics - Wheels/4(ω), Quaternion Dynamics/1(ω)
  Ωₓ/1 -> Reaction Wheels Dynamics/1(Ωₓ), Angular Velocity Dynamics - Wheels/1(Ωₓ)
  q/1 -> Quaternion Dynamics/2(q)
  Quaternion Dynamics/1(dq/dt) -> dq/dt/1
  Mᵣ/1 -> Reaction Wheels Dynamics/2(Mᵣ)
  Iᵣ Inv/1 -> Reaction Wheels Dynamics/3(Iᵣ Inv)
  Reaction Wheels Dynamics/1(dωᵣ/dt) -> dωᵣ/dt/1
  RIᵣ/1 -> Reaction Wheels Dynamics/4(RIᵣ)
  Reaction Wheels Dynamics/2(Wheels) -> Angular Velocity Dynamics - Wheels/6(Wheels)
  ωᵣ/1 -> Reaction Wheels Dynamics/5(ωᵣ)

== system DKE_Library/Attitude Dynamics -  Wheels/Matrix Assembly ==
  note: [kgm²]
  note: [1/kgm²]
  note: [1/kgm²]
  note: [kgm²]
  note: [rad/s]
  "ω " : Inport
  Iₘ : Constant  Value=I
  MatrixMultiply : Product  Multiplication=Matrix(*)
  "RIᵣ  " : Constant  Value=RW.AI
  RW Mounting Error : Constant  Value=RW.MountErr
  Skew Symmetric Matrix : MATH_library/Skew Symmetric Matrix
  "inv Iᵣ  " : Constant  Value=1/RW.I
  inv Iₘ : Constant  Value=invI
  "Iₘ " : Outport  VectorParamsAs1DForOutWhenUnconnected=off
  Ωₓ : Outport  Port=2  VectorParamsAs1DForOutWhenUnconnected=off
  Iₘ inv : Outport  Port=3  VectorParamsAs1DForOutWhenUnconnected=off
  Iᵣ inv : Outport  Port=4  VectorParamsAs1DForOutWhenUnconnected=off
  RIᵣ : Outport  Port=5  VectorParamsAs1DForOutWhenUnconnected=off
  wires:
  inv Iₘ/1 -> Iₘ inv/1
  Iₘ/1 -> "Iₘ "/1
  "ω "/1 -> Skew Symmetric Matrix/1
  Skew Symmetric Matrix/1 -> Ωₓ/1
  "inv Iᵣ  "/1 -> Iᵣ inv/1
  MatrixMultiply/1 -> RIᵣ/1
  "RIᵣ  "/1 -> MatrixMultiply/2
  RW Mounting Error/1 -> MatrixMultiply/1

== system DKE_Library/Attitude Dynamics -  Wheels/Wheels Sat. ==
  note: Each element in the output vector is true
      | if the corresponding wheel is saturated.
  ωᵣ : Inport
  Abs : Abs
  Compare To Constant : simulink/Logic and Bit Operations/Compare To Constant  relop=>=  const=0.999*RW.MaxWheelW  OutDataTypeStr=boolean
  Sat. : Outport  VectorParamsAs1DForOutWhenUnconnected=off
  wires:
  ωᵣ/1 -> Abs/1
  Abs/1 -> Compare To Constant/1
  Compare To Constant/1 -> Sat./1

== system DKE_Library/Attitude Dynamics - No Wheels/Derivatives ==
  q : Inport
  Iₘ : Inport  Port=2
  Ωₓ : Inport  Port=3
  Iₘ Inv : Inport  Port=4
  ω : Inport  Port=5
  tₚ : Inport  Port=6
  Angular Velocity Dynamics : Subsystem
  Quaternion Dynamics : Subsystem
  dq/dt : Outport  VectorParamsAs1DForOutWhenUnconnected=off
  dω/dt : Outport  Port=2  VectorParamsAs1DForOutWhenUnconnected=off
  wires:
  tₚ/1 -> Angular Velocity Dynamics/5(tₚ)
  Iₘ Inv/1 -> Angular Velocity Dynamics/3(Iₘ Inv)
  Angular Velocity Dynamics/1(dω/dt) -> dω/dt/1
  Iₘ/1 -> Angular Velocity Dynamics/2(Iₘ)
  ω/1 -> Angular Velocity Dynamics/4(ω), Quaternion Dynamics/1(ω)
  Ωₓ/1 -> Angular Velocity Dynamics/1(Ωₓ)
  q/1 -> Quaternion Dynamics/2(q)
  Quaternion Dynamics/1(dq/dt) -> dq/dt/1

== system DKE_Library/Attitude Dynamics - No Wheels/Matrix Assembly ==
  note: [1/kgm²]
  note: [kgm²]
  note: [rad/s]
  "ω " : Inport
  Iₘ : Constant  Value=I
  Skew Symmetric Matrix : MATH_library/Skew Symmetric Matrix
  invIₘ : Constant  Value=invI
  "Iₘ " : Outport  VectorParamsAs1DForOutWhenUnconnected=off
  Ωₓ : Outport  Port=2  VectorParamsAs1DForOutWhenUnconnected=off
  Iₘ inv : Outport  Port=3  VectorParamsAs1DForOutWhenUnconnected=off
  wires:
  invIₘ/1 -> Iₘ inv/1
  Iₘ/1 -> "Iₘ "/1
  "ω "/1 -> Skew Symmetric Matrix/1
  Skew Symmetric Matrix/1 -> Ωₓ/1

== system DKE_Library/ECI2LVLH RotMat/Rotation Matrices ==
  pos : Inport
  vel : Inport  Port=2
  Constant : Constant  Value=0
  Constant1 : Constant  Value=0
  Gain : Gain  Gain=-1
  MatrixMultiply : Product  Multiplication=Matrix(*)
  Mean Motion : Subsystem
  Skew Symmetric Matrix : MATH_library/Skew Symmetric Matrix
  Vector Concatenate : Concatenate  NumInputs=3
  XY to DCM : MATH_library/XY to DCM
  DCM : Outport  VectorParamsAs1DForOutWhenUnconnected=off
  dDCM : Outport  Port=2  VectorParamsAs1DForOutWhenUnconnected=off
  wires:
  vel/1 -> Mean Motion/2(vel), XY to DCM/2
  pos/1 -> Mean Motion/1(pos), XY to DCM/1
  XY to DCM/1 -> MatrixMultiply/1, DCM/1
  Constant1/1 -> Vector Concatenate/2
  Constant/1 -> Vector Concatenate/1
  Mean Motion/1(n) -> Vector Concatenate/3
  Vector Concatenate/1 -> Skew Symmetric Matrix/1
  Skew Symmetric Matrix/1 -> MatrixMultiply/2
  MatrixMultiply/1 -> Gain/1
  Gain/1 -> dDCM/1

== system DKE_Library/Environment Perturbations/Drag Perturbation ==
  note: [Nm]
  note: [m/s²]
  note: [m/s]
  note: [m]
  note: [rad/s]
  r_sat : Inport
  A : Inport  Port=2
  v_sat : Inport  Port=3
  ω : Inport  Port=4
  Air Density : ENV_Library/Air Density  RBODY=RADIUS_EARTH  rho_h=rho_h
  Drag Faces : ENV_Library/Drag Faces  CD=CD  m=mass  NS=NS  S_faces=S_faces  N_faces=N_faces  R_faces=R_faces
  a_drag : Outport  VectorParamsAs1DForOutWhenUnconnected=off
  t_drag : Outport  Port=2  VectorParamsAs1DForOutWhenUnconnected=off
  wires:
  v_sat/1 -> Drag Faces/2
  Drag Faces/2 -> t_drag/1
  Drag Faces/1 -> a_drag/1
  ω/1 -> Drag Faces/4
  r_sat/1 -> Drag Faces/1, Air Density/1
  Air Density/1 -> Drag Faces/5
  A/1 -> Drag Faces/3

== system DKE_Library/Environment Perturbations/Gravity Perturbations ==
  note: [m/s²]
  note: [m]
  note: [m]
  note: [m]
  note: [Nm]
  r_sat : Inport
  r_sun : Inport  Port=2
  r_moon : Inport  Port=3
  A : Inport  Port=4
  Iₘ : Inport  Port=5
  R_ecef2eci : Inport  Port=6
  Gravity Gradient : ENV_Library/Gravity Gradient  GM=GM_EARTH
  Gravity Spherical Harmonics : ENV_Library/Gravity Spherical Harmonics  GRAV=grav_data
  Moon's Pertubation : ENV_Library/Third Body Acceleration  GM=GM_MOON
  Subtract : Sum  Inputs=+++
  Sun's Perturbation : ENV_Library/Third Body Acceleration  GM=GM_SUN
  a_grav : Outport  VectorParamsAs1DForOutWhenUnconnected=off
  t_grav : Outport  Port=2  VectorParamsAs1DForOutWhenUnconnected=off
  wires:
  R_ecef2eci/1 -> Gravity Spherical Harmonics/2
  A/1 -> Gravity Gradient/2
  Iₘ/1 -> Gravity Gradient/3
  r_sun/1 -> Sun's Perturbation/2
  r_sat/1 -> Gravity Spherical Harmonics/1, Sun's Perturbation/1, Gravity Gradient/1, Moon's Pertubation/1
  Sun's Perturbation/1 -> Subtract/2
  r_moon/1 -> Moon's Pertubation/2
  Moon's Pertubation/1 -> Subtract/3
  Gravity Gradient/1 -> t_grav/1
  Subtract/1 -> a_grav/1
  Gravity Spherical Harmonics/1 -> Subtract/1

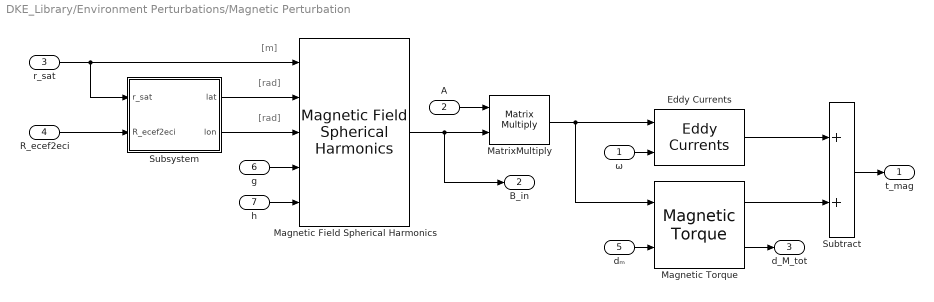
== system DKE_Library/Environment Perturbations/Magnetic Perturbation ==
  note: [rad]
  note: [m]
  note: [rad]
  ω : Inport
  A : Inport  Port=2
  r_sat : Inport  Port=3
  R_ecef2eci : Inport  Port=4
  dₘ : Inport  Port=5
  g : Inport  Port=6
  h : Inport  Port=7
  Eddy Currents : ENV_Library/Eddy Currents  Ke=Keddy
  "Magnetic Field Spherical Harmonics  " : ENV_Library/Magnetic Field  Spherical Harmonics    mag_data=mag_data
  Magnetic Torque : ENV_Library/Magnetic Torque  parasitic=paras_dipole
  MatrixMultiply : Product  Multiplication=Matrix(*)
  Subsystem : Subsystem
  Subtract : Sum
  t_mag : Outport  VectorParamsAs1DForOutWhenUnconnected=off
  B_in : Outport  Port=2  VectorParamsAs1DForOutWhenUnconnected=off
  d_M_tot : Outport  Port=3  VectorParamsAs1DForOutWhenUnconnected=off
  wires:
  r_sat/1 -> "Magnetic Field Spherical Harmonics  "/1, Subsystem/1(r_sat)
  Eddy Currents/1 -> Subtract/1
  g/1 -> "Magnetic Field Spherical Harmonics  "/4
  dₘ/1 -> Magnetic Torque/2
  ω/1 -> Eddy Currents/2
  Magnetic Torque/1 -> Subtract/2
  Subtract/1 -> t_mag/1
  MatrixMultiply/1 -> Magnetic Torque/1, Eddy Currents/1
  A/1 -> MatrixMultiply/1
  "Magnetic Field Spherical Harmonics  "/1 -> B_in/1, MatrixMultiply/2
  R_ecef2eci/1 -> Subsystem/2(R_ecef2eci)
  Subsystem/1(lat) -> "Magnetic Field Spherical Harmonics  "/2
  Subsystem/2(lon) -> "Magnetic Field Spherical Harmonics  "/3
  Magnetic Torque/2 -> d_M_tot/1
  h/1 -> "Magnetic Field Spherical Harmonics  "/5

== system DKE_Library/Environment Perturbations/SRP Perturbation ==
  note: [m]
  note: [m/s²]
  note: [Nm]
  note: [m]
  r_sat : Inport
  r_sun : Inport  Port=2
  A : Inport  Port=3
  Add : Sum  Inputs=-+
  Cast To Double : DataTypeConversion  OutDataTypeStr=double
  Compare To Constant : simulink/Logic and Bit Operations/Compare To Constant  relop===  const=1.0  OutDataTypeStr=boolean
  Constant : Constant
  SRP Faces : ENV_Library/SRP Faces   m=mass  c_dif=c_dif  c_spe=c_spe  NS=NS  S_faces=S_faces  N_faces=N_faces  R_faces=R_faces
  Shadow Function : ENV_Library/Shadow Function   Rsun=RADIUS_SUN  Rbody=RADIUS_EARTH+ATMO_HEIGHT
  a_srp : Outport  VectorParamsAs1DForOutWhenUnconnected=off
  t_srp : Outport  Port=2  VectorParamsAs1DForOutWhenUnconnected=off
  cth : Outport  Port=3  VectorParamsAs1DForOutWhenUnconnected=off
  Albedo : Outport  Port=4  VectorParamsAs1DForOutWhenUnconnected=off
  Eclipse : Outport  Port=5  VectorParamsAs1DForOutWhenUnconnected=off
  wires:
  A/1 -> SRP Faces/3
  Shadow Function/1 -> SRP Faces/4, Add/1, Compare To Constant/1
  SRP Faces/1 -> a_srp/1
  r_sat/1 -> SRP Faces/1, Shadow Function/1
  SRP Faces/2 -> t_srp/1
  r_sun/1 -> SRP Faces/2, Shadow Function/2
  SRP Faces/3 -> cth/1
  Compare To Constant/1 -> Cast To Double/1
  Add/1 -> Eclipse/1
  Constant/1 -> Add/2
  Cast To Double/1 -> Albedo/1

== system DKE_Library/Kinematics/Inertial to Perifocal ==
  note: [rad]
  note: [rad]
  note: [rad]
  inc : Inport
  ran : Inport  Port=2
  aop : Inport  Port=3
  Rotation Angles to Direction Cosine Matrix : sharedtransform/Rotation Angles to Direction Cosine Matrix  rotationOrder=ZXZ  aMode=aMode
      settings: SourceProductBaseCode=AE,PW,DR,MT,UV,VE
  Vector Concatenate1 : Concatenate  NumInputs=3
  R : Outport  VectorParamsAs1DForOutWhenUnconnected=off
  wires:
  Rotation Angles to Direction Cosine Matrix/1 -> R/1
  inc/1 -> Vector Concatenate1/2
  Vector Concatenate1/1 -> Rotation Angles to Direction Cosine Matrix/1
  ran/1 -> Vector Concatenate1/1
  aop/1 -> Vector Concatenate1/3

== system DKE_Library/car2coe/Eccentricity ==
  h : Inport
  u_pos : Inport  Port=2
  vel : Inport  Port=3
  Add : Sum  Inputs=+-
  Cross Product : MATH_library/Cross Product
  Gain : Gain  Gain=1/GM  OutDataTypeStr=Inherit: Same as input
  Normalise & Norm : MATH_library/Normalise & Norm
  ecc : Outport  VectorParamsAs1DForOutWhenUnconnected=off
  e_vect : Outport  Port=2  VectorParamsAs1DForOutWhenUnconnected=off
  wires:
  Normalise & Norm/2 -> ecc/1
  Add/1 -> Normalise & Norm/1
  Normalise & Norm/1 -> e_vect/1
  vel/1 -> Cross Product/1
  h/1 -> Cross Product/2
  Cross Product/1 -> Gain/1
  Gain/1 -> Add/1
  u_pos/1 -> Add/2

== system DKE_Library/car2coe/Inclination ==
  h : Inport
  Divide : Product  Inputs=*/  OutDataTypeStr=Inherit: Same as first input
  Saturation : Saturate  UpperLimit=1  LowerLimit=-1
  Selector : Selector  InputPortWidth=3  IndexOptions=Index vector (dialog)  Indices=3  OutputSizes=1
  Trigonometric Function : Trigonometry  Operator=acos  OutputSignalType=real
  Vector Norm : MATH_library/Vector Norm
  inc : Outport  VectorParamsAs1DForOutWhenUnconnected=off
  wires:
  Saturation/1 -> Trigonometric Function/1
  Trigonometric Function/1 -> inc/1
  Vector Norm/1 -> Divide/2
  h/1 -> Vector Norm/1, Selector/1
  Selector/1 -> Divide/1
  Divide/1 -> Saturation/1

== system DKE_Library/car2coe/LineNodes ==
  h : Inport
  Constant : Constant  Value=[0 0 1]  OutDataTypeStr=Inherit: Inherit via back propagation
  Cross Product : MATH_library/Cross Product
  Normalise : MATH_library/Normalise
  N : Outport  VectorParamsAs1DForOutWhenUnconnected=off
  wires:
  Cross Product/1 -> Normalise/1
  h/1 -> Cross Product/2
  Constant/1 -> Cross Product/1
  Normalise/1 -> N/1

== system DKE_Library/car2coe/Normalize1 ==
  pos : Inport
  Normalise & Norm : MATH_library/Normalise & Norm
  Reciprocal : Product  Inputs=/
  inv_r : Outport  VectorParamsAs1DForOutWhenUnconnected=off
  u_pos : Outport  Port=2  VectorParamsAs1DForOutWhenUnconnected=off
  wires:
  Normalise & Norm/1 -> u_pos/1
  Reciprocal/1 -> inv_r/1
  pos/1 -> Normalise & Norm/1
  Normalise & Norm/2 -> Reciprocal/1

== system DKE_Library/car2coe/PericenterAnomaly ==
  e_vect : Inport
  N : Inport  Port=2
  Add : Sum  Inputs=-+  OutDataTypeStr=Inherit: Same as first input
  Constant : Constant  Value=2*pi  OutDataTypeStr=Inherit: Inherit via back propagation
  Dot Product : DotProduct  InputSameDT=on
  Saturation : Saturate  UpperLimit=1  LowerLimit=-1
  Selector : Selector  InputPortWidth=3  IndexOptions=Index vector (dialog)  Indices=3  OutputSizes=1
  Switch : Switch  Criteria=u2 > Threshold
  Trigonometric Function : Trigonometry  Operator=acos  OutputSignalType=real
  aop : Outport  VectorParamsAs1DForOutWhenUnconnected=off
  wires:
  Saturation/1 -> Trigonometric Function/1
  N/1 -> Dot Product/1
  e_vect/1 -> Selector/1, Dot Product/2
  Selector/1 -> Switch/2
  Dot Product/1 -> Saturation/1
  Switch/1 -> aop/1
  Trigonometric Function/1 -> Switch/1, Add/1
  Add/1 -> Switch/3
  Constant/1 -> Add/2

== system DKE_Library/car2coe/RAAN ==
  N : Inport
  Demux : Demux  Outputs=2
  Selector : Selector  InputPortWidth=3  IndexOptions=Index vector (dialog)  Indices=[2 1]  OutputSizes=1
  Trigonometric Function : Trigonometry  Operator=atan2  OutputSignalType=real
  ran : Outport  VectorParamsAs1DForOutWhenUnconnected=off
  wires:
  Demux/1 -> Trigonometric Function/1
  Demux/2 -> Trigonometric Function/2
  Selector/1 -> Demux/1
  Trigonometric Function/1 -> ran/1
  N/1 -> Selector/1

== system DKE_Library/car2coe/SemiMajorAxis ==
  inv_r : Inport
  vel : Inport  Port=2
  Add : Sum  Inputs=-+
  Dot Product : DotProduct  InputSameDT=on  OutDataTypeStr=Inherit: Inherit via internal rule
  Gain : Gain  Gain=GM  OutDataTypeStr=Inherit: Same as input
  Gain1 : Gain  Gain=0.5  OutDataTypeStr=single
  Gain2 : Gain  Gain=-GM/2  OutDataTypeStr=Inherit: Same as input
  Reciprocal : Product  Inputs=/
  sma : Outport  VectorParamsAs1DForOutWhenUnconnected=off
  wires:
  Reciprocal/1 -> Gain2/1
  vel/1 -> Dot Product/2, Dot Product/1
  inv_r/1 -> Gain/1
  Dot Product/1 -> Gain1/1
  Gain/1 -> Add/1
  Gain1/1 -> Add/2
  Add/1 -> Reciprocal/1
  Gain2/1 -> sma/1

== system DKE_Library/car2coe/TrueAnomaly ==
  u_pos : Inport
  vel : Inport  Port=2
  e_vect : Inport  Port=3
  Add : Sum  Inputs=-+  OutDataTypeStr=Inherit: Same as first input
  Constant : Constant  Value=2*pi  OutDataTypeStr=Inherit: Inherit via back propagation
  Dot Product : DotProduct  InputSameDT=on
  Dot Product1 : DotProduct  InputSameDT=on
  Saturation : Saturate  UpperLimit=1  LowerLimit=-1
  Switch : Switch  Criteria=u2 > Threshold
  Trigonometric Function : Trigonometry  Operator=acos  OutputSignalType=real
  th : Outport  VectorParamsAs1DForOutWhenUnconnected=off
  wires:
  Saturation/1 -> Trigonometric Function/1
  Add/1 -> Switch/3
  vel/1 -> Dot Product1/1
  Constant/1 -> Add/2
  Trigonometric Function/1 -> Switch/1, Add/1
  Switch/1 -> th/1
  Dot Product/1 -> Saturation/1
  Dot Product1/1 -> Switch/2  "radial velocity"
  u_pos/1 -> Dot Product/1, Dot Product1/2
  e_vect/1 -> Dot Product/2

== system DKE_Library/ Simple Thermal Models/Earth_view_factor /Vector Cos Angle w.r.t S//C Faces ==
  vect : Inport
  Normalise : MATH_library/Normalise
  Product4 : Product  Multiplication=Matrix(*)
  Reshape2 : Reshape  OutputDimensionality=Row vector (2-D)
  Surf Axis in principal Inertia is the normal direction. : Constant  Value=N_surf
  cos_f : Outport  VectorParamsAs1DForOutWhenUnconnected=off
  wires:
  Product4/1 -> cos_f/1
  Normalise/1 -> Reshape2/1
  Reshape2/1 -> Product4/1
  vect/1 -> Normalise/1
  Surf Axis in principal Inertia is the normal direction./1 -> Product4/2

== system DKE_Library/Attitude Dynamics -  Wheels/Derivatives/Angular Velocity Dynamics - Wheels ==
  note: The ' Wheels ' contribution includes all the terms coming from the
      | reaction wheels that enter the global spacecraft dynamic equation.
  Ωₓ : Inport
  Iₘ : Inport  Port=2
  Iₘ Inv : Inport  Port=3
  ω : Inport  Port=4
  Mₚ : Inport  Port=5
  Wheels : Inport  Port=6
  Add : Sum  Inputs=+--
  Product : Product  Multiplication=Matrix(*)
  Product1 : Product  Multiplication=Matrix(*)
  Product2 : Product  Multiplication=Matrix(*)
  dω/dt : Outport  VectorParamsAs1DForOutWhenUnconnected=off
  wires:
  Product2/1 -> dω/dt/1
  Iₘ Inv/1 -> Product2/1
  Add/1 -> Product2/2
  Product1/1 -> Add/2
  Product/1 -> Product1/2
  Ωₓ/1 -> Product1/1
  Iₘ/1 -> Product/1
  ω/1 -> Product/2
  Mₚ/1 -> Add/1
  Wheels/1 -> Add/3

== system DKE_Library/Attitude Dynamics -  Wheels/Derivatives/Quaternion Dynamics ==
  ω : Inport
  q : Inport  Port=2
  Gain2 : Gain  Gain=0.5
  Product : Product  Multiplication=Matrix(*)
  Ω Matrix : Subsystem
  dq/dt : Outport  VectorParamsAs1DForOutWhenUnconnected=off
  wires:
  Ω Matrix/1(Ω) -> Gain2/1
  Gain2/1 -> Product/1
  ω/1 -> Ω Matrix/1(ω)
  Product/1 -> dq/dt/1
  q/1 -> Product/2

== system DKE_Library/Attitude Dynamics -  Wheels/Derivatives/Reaction Wheels Dynamics ==
  note: The second contribution to the ' Wheels ' term is the coupling between
      | the spacecraft angular velocity and the wheels angular momentum
  Ωₓ : Inport
  Mᵣ : Inport  Port=2
  Iᵣ Inv : Inport  Port=3
  RIᵣ : Inport  Port=4
  ωᵣ : Inport  Port=5
  MatrixMultiply : Product
  MatrixMultiply1 : Product  Multiplication=Matrix(*)
  MatrixMultiply2 : Product  Inputs=3  Multiplication=Matrix(*)
  Subtract : Sum
  dωᵣ/dt : Outport  VectorParamsAs1DForOutWhenUnconnected=off
  Wheels : Outport  Port=2  VectorParamsAs1DForOutWhenUnconnected=off
  wires:
  Iᵣ Inv/1 -> MatrixMultiply/1
  Mᵣ/1 -> MatrixMultiply/2
  MatrixMultiply/1 -> MatrixMultiply1/2, dωᵣ/dt/1
  RIᵣ/1 -> MatrixMultiply2/2, MatrixMultiply1/1
  MatrixMultiply1/1 -> Subtract/1
  MatrixMultiply2/1 -> Subtract/2
  Subtract/1 -> Wheels/1
  Ωₓ/1 -> MatrixMultiply2/1
  ωᵣ/1 -> MatrixMultiply2/3

== system DKE_Library/Attitude Dynamics - No Wheels/Derivatives/Angular Velocity Dynamics ==
  Ωₓ : Inport
  Iₘ : Inport  Port=2
  Iₘ Inv : Inport  Port=3
  ω : Inport  Port=4
  tₚ : Inport  Port=5
  Add : Sum  Inputs=+-
  Product : Product  Multiplication=Matrix(*)
  Product1 : Product  Multiplication=Matrix(*)
  Product2 : Product  Multiplication=Matrix(*)
  dω/dt : Outport  VectorParamsAs1DForOutWhenUnconnected=off
  wires:
  Product2/1 -> dω/dt/1
  Iₘ Inv/1 -> Product2/1
  Add/1 -> Product2/2
  Product1/1 -> Add/2
  Product/1 -> Product1/2
  Ωₓ/1 -> Product1/1
  Iₘ/1 -> Product/1
  ω/1 -> Product/2
  tₚ/1 -> Add/1

== system DKE_Library/Attitude Dynamics - No Wheels/Derivatives/Quaternion Dynamics ==
  ω : Inport
  q : Inport  Port=2
  Gain2 : Gain  Gain=0.5
  Product : Product  Multiplication=Matrix(*)
  Ω Matrix : Subsystem
  dq/dt : Outport  VectorParamsAs1DForOutWhenUnconnected=off
  wires:
  Ω Matrix/1(Ω) -> Gain2/1
  Gain2/1 -> Product/1
  ω/1 -> Ω Matrix/1(ω)
  Product/1 -> dq/dt/1
  q/1 -> Product/2

== system DKE_Library/ECI2LVLH RotMat/Rotation Matrices/Mean Motion ==
  pos : Inport
  vel : Inport  Port=2
  Constant : Constant  Value=3
  Constant1 : Constant  Value=GM
  Divide : Product  Inputs=/*
  Pow : Math  Operator=pow  RndMeth=Zero  SaturateOnIntegerOverflow=on
  Reciprocal : Product  Inputs=/
  SemiMajorAxis : $bdroot/car2coe/SemiMajorAxis  SystemSampleTime=-1  Latency=0  AutoFrameSizeCalculation=off
  Sqrt : Sqrt  SaturateOnIntegerOverflow=on
  Vector Norm : MATH_library/Vector Norm
  n : Outport  VectorParamsAs1DForOutWhenUnconnected=off
  wires:
  Pow/1 -> Divide/1
  Vector Norm/1 -> Reciprocal/1
  Divide/1 -> Sqrt/1
  Constant1/1 -> Divide/2
  vel/1 -> SemiMajorAxis/2
  Constant/1 -> Pow/2
  SemiMajorAxis/1 -> Pow/1
  Sqrt/1 -> n/1
  Reciprocal/1 -> SemiMajorAxis/1
  pos/1 -> Vector Norm/1

== system DKE_Library/Environment Perturbations/Magnetic Perturbation/Subsystem ==
  note: [rad]
  note: [m]
  note: [rad]
  r_sat : Inport
  R_ecef2eci : Inport  Port=2
  Cartesian to Spherical : ENV_Library/Cartesian to Spherical
  MatrixMultiply1 : Product  Multiplication=Matrix(*)
  Terminator : Terminator
  Transpose : Math  Operator=transpose  SaturateOnIntegerOverflow=on
  lat : Outport  VectorParamsAs1DForOutWhenUnconnected=off
  lon : Outport  Port=2  VectorParamsAs1DForOutWhenUnconnected=off
  wires:
  Cartesian to Spherical/1 -> lat/1
  Cartesian to Spherical/2 -> lon/1
  Transpose/1 -> MatrixMultiply1/1
  r_sat/1 -> MatrixMultiply1/2
  R_ecef2eci/1 -> Transpose/1
  MatrixMultiply1/1 -> Cartesian to Spherical/1
  Cartesian to Spherical/3 -> Terminator/1

== system DKE_Library/Attitude Dynamics -  Wheels/Derivatives/Quaternion Dynamics/Ω Matrix ==
  ω : Inport
  Add : Sum  Inputs=+++
  Demux : Demux  Outputs=3
  Gain1 : Gain  Gain=[0 0 -1 0; 0 0 0 1; 1 0 0 0; 0 -1 0 0]
  Gain3 : Gain  Gain=[0 1 0 0; -1 0 0 0; 0 0 0 1; 0 0 -1 0]
  Gain4 : Gain  Gain=[0 0 0 1; 0 0 1 0; 0 -1 0 0; -1 0 0 0]
  Ω : Outport  VectorParamsAs1DForOutWhenUnconnected=off
  wires:
  ω/1 -> Demux/1
  Gain1/1 -> Add/2
  Gain3/1 -> Add/3
  Gain4/1 -> Add/1
  Demux/2 -> Gain1/1
  Demux/3 -> Gain3/1
  Add/1 -> Ω/1
  Demux/1 -> Gain4/1
